simulink model "apf_simulink"  (R2023a)
settings: Solver=VariableStepAuto  StartTime=0.0  StopTime=1  RelTol=1e-3
libraries: simulink x2
settings Model: Creator=andykim02  LastModifiedBy=andykim02
settings SFSimCC: SimCustomHeaderCode="#include \"APF.h\""  SimUserSources=apf.c

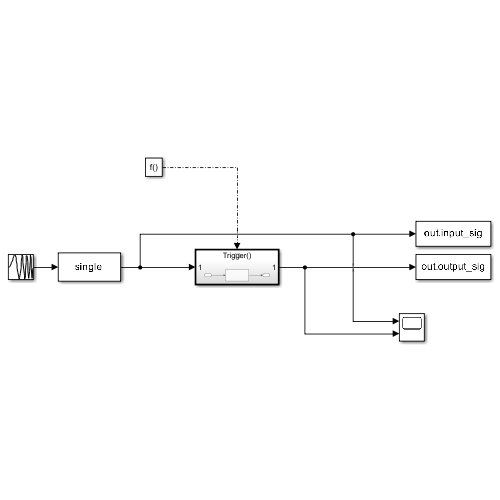
[thumbnail: Simulink's stored preview of the top-level diagram]
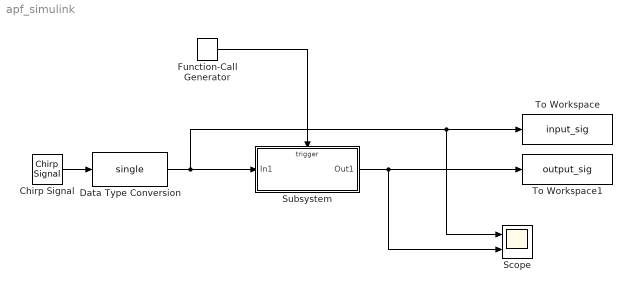
== system apf_simulink ==
  Chirp Signal : simulink/Sources/Chirp Signal  f1=10  T=1  f2=1000
  Data Type Conversion : DataTypeConversion  OutDataTypeStr=single  SaturateOnIntegerOverflow=off  RndMeth=Floor
  Function-Call Generator : simulink/Ports & Subsystems/Function-Call Generator  sample_time=1e-4  numberOfIterations=1  DisallowWideOutput=off
  Scope : Scope  NumInputPorts=2
  Subsystem : Subsystem
  To Workspace : ToWorkspace  VariableName=input_sig  SampleTime=-1
  To Workspace1 : ToWorkspace  VariableName=output_sig  SampleTime=-1
  wires:
  Subsystem/1(Out1) -> To Workspace1/1, Scope/2
  Chirp Signal/1 -> Data Type Conversion/1
  Function-Call Generator/1 -> Subsystem/Trigger
  Data Type Conversion/1 -> To Workspace/1, Scope/1, Subsystem/1(In1)

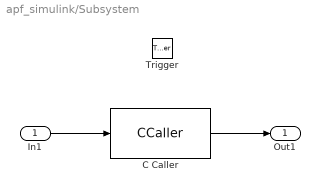
== system apf_simulink/Subsystem ==
  In1 : Inport
  Trigger : TriggerPort  TriggerType=function-call  VariantControl=(inherit)  PortDimensions=1
  C Caller : CCaller  FunctionName=APF_Update  PortSpecificationStruct="%)30     .    N ,   8    (     @         %    \"     (    !     0         %  0 \"0    $    _    07)G3F%M90  4&]R=$YA;64 4V-O<&4     26YD97@     5'EP90      4VEZ90      27-';&]B86P   X    P    !@    @    $          4    (     0    ,    !         !   P!O=70 #@   #     &    \"     0         !0    @    !     P    $         $  # &]U=  .    .     8    (    !          %    \"     $    &     0         0    !@   $]U='!U=   #@   #@    &    \"     8         !0    @    !     0    $         \"0    @               X    X    !@    @    $          4    (     0    8    !         !     &    <VEN9VQE   .    ,     8    (    !          %    \"     $    !     0         0  $ ,0    X    P    !@    @    ) @        4    (     0    $    !          (  0      #@   #     &    \"     0         !0    @    !     0    $         $  ! '@    .    ,     8    (    !          %    \"     $    !     0         0  $ >     X    X    !@    @    $          4    (     0    4    !         !     %    26YP=70    .    .     8    (    !@         %    \"     $    !     0         )    \"               #@   #@    &    \"     0         !0    @    !    !@    $         $     8   !S:6YG;&4   X    P    !@    @    $          4    (     0    $    !         !   0 Q    #@   #     &    \"     D\"        !0    @    !     0    $          @ !"
  Out1 : Outport
  wires:
  In1/1 -> C Caller/1
  C Caller/1 -> Out1/1
